simulink model "OBSERVER1"  (R2020a)
settings: Solver=VariableStepAuto  StartTime=0.0  StopTime=10  RelTol=1e-3
values from neighbouring files (symbols this model uses):
  A = [0 1 0;0 0 1;-15 -23 -9]    [cau1.m]    (also in cau2.m = [0 1 0;0 0 1;-2 -5 -4])
  Aobs = [A-L*C]    [cau1.m]    (also in cau2.m)
  B = [0;0;1]    [cau1.m]    (also in cau2.m = [-7;19;-43])
  Bobs = [B-L*D L]    [cau1.m]    (also in cau2.m)
  C = [-13.5 -18.25 -5]    [cau1.m]    (also in cau2.m = [1 0 0])
  Cobs = eye(3)    [cau1.m]    (also in cau2.m)
  D = 1    [cau1.m]    (also in cau2.m = 0)
  Dobs = zeros(3,2)    [cau1.m]    (also in cau2.m)
settings Model: Creator=ngtuan  LastModifiedBy=ngtuan

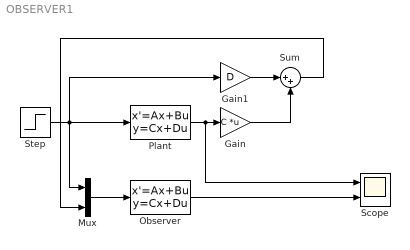
== system OBSERVER1 ==
  Gain : Gain  Gain=C  Multiplication=Matrix(K*u)
  Gain1 : Gain  Gain=D
  Mux : Mux  Inputs=2
  Observer : StateSpace  A=Aobs  B=Bobs  C=Cobs  D=Dobs  InitialCondition=0
  Plant : StateSpace  A=A  B=B  C=eye(3)  D=[0;0;0]  InitialCondition=0
  Scope : Scope  NumInputPorts=2
  Step : Step  Time=0  SampleTime=0
  Sum : Sum  Inputs=|++
  wires:
  Step/1 -> Gain1/1, Mux/1, Plant/1
  Mux/1 -> Observer/1
  Plant/1 -> Scope/1, Gain/1
  Sum/1 -> Mux/2
  Gain1/1 -> Sum/1
  Gain/1 -> Sum/2
  Observer/1 -> Scope/2
